simulink model "ControlSystem"  (R2026a)
settings: Solver=FixedStepDiscrete  FixedStep=1/200
undefined symbols (not defined in the file or in its folder): control, position, reversible_flags, timestamp, timestamp_sample, velocity
libraries: px4_lib x31
settings Model: Creator=jack  LastModifiedBy=jack
settings OptimizationCC: DefaultUnderspecifiedDataType=single
settings DebuggingCC: ParameterPrecisionLossMsg=none  UnnecessaryDatatypeConvMsg=warning
settings HardwareCC: ProdBitPerLong=64.0  ProdHWDeviceType=Intel->x86-64 (Linux 64)
settings SFSimCC: SimCustomHeaderCode="#include \"px4_simulink_api.h\""  SimUserSources=px4_simulink_api.cpp  SimTargetLang=C++
settings RTWCC: SystemTargetFile=ert.tlc  GenCodeOnly=on  PostCodeGenCommand=px4io.px4API.runPostCodeGen(buildInfo)  CustomHeaderCode="#include \"px4_simulink_api.h\""  DataTypeReplacement=CDataTypesFixedWidth  TargetLang=C++  Description=Embedded Coder
settings ERTTargetCC: ExtModeTransport=2.0  RootIOFormat=Structure reference  MaxIdInt64=INT64_MAX  MinIdInt64=INT64_MIN  MaxIdUint64=UINT64_MAX  MaxIdInt32=INT32_MAX  MinIdInt32=INT32_MIN  MaxIdUint32=UINT32_MAX  MaxIdInt16=INT16_MAX  MinIdInt16=INT16_MIN  MaxIdUint16=UINT16_MAX  MaxIdInt8=INT8_MAX  MinIdInt8=INT8_MIN  MaxIdUint8=UINT8_MAX  TargetLangStandard=C++14 (ISO)  CodeInterfacePackaging=C++ class  SubcomponentCodeInterfacePackaging=C++ class  ParenthesesLevel=Standards  CastingMode=Standards

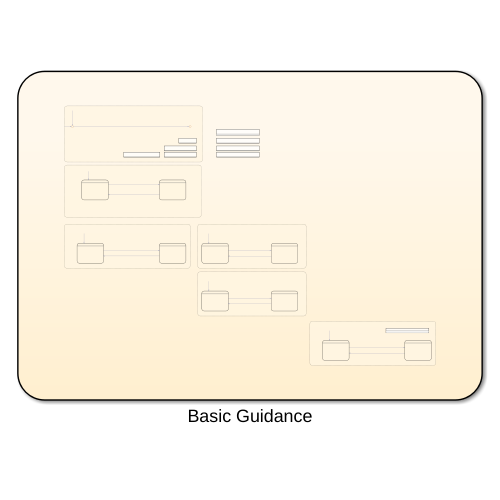
[thumbnail: Simulink's stored preview of the top-level diagram]
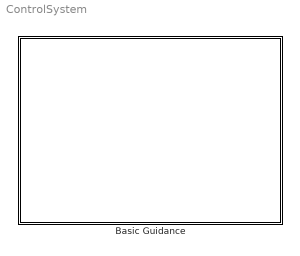
== system ControlSystem ==
  Basic Guidance : Stateflow chart  TreatAsAtomicUnit=on

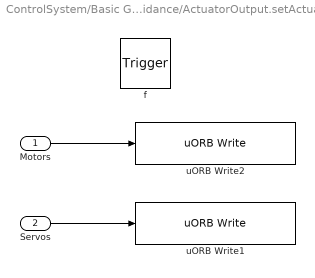
== system ControlSystem/Basic Guidance/ActuatorOutput.setActuators ==
  Motors : Inport  OutDataTypeStr=Bus: actuator_motors_s  PortDimensions=1
  Servos : Inport  Port=2  OutDataTypeStr=Bus: actuator_servos_s  PortDimensions=1
  f : TriggerPort  TriggerType=function-call  VariantControl=(inherit)
      settings: CopyFcn=Stateflow.SLINSF.SimulinkMan.removeBlockPreDeleteFcn  PreDeleteFcn=Stateflow.SLINSF.SimulinkMan.unsafePredeleteFcn
  uORB Write1 : px4_lib/uORB Write  uorb_topic=actuator_servos  uorb_variant=actuator_servos  sample_time=-1
  uORB Write2 : px4_lib/uORB Write  uorb_topic=actuator_motors  uorb_variant=actuator_motors  sample_time=-1
  wires:
  Motors/1 -> uORB Write2/1
  Servos/1 -> uORB Write1/1

== system ControlSystem/Basic Guidance/GuidanceRequestUpdate.Update.setGuidanceRequest ==
  GuidanceRequest : Inport  OutDataTypeStr=Bus: sim_guidance_request_s  PortDimensions=1
  f : TriggerPort  TriggerType=function-call  VariantControl=(inherit)
      settings: CopyFcn=Stateflow.SLINSF.SimulinkMan.removeBlockPreDeleteFcn  PreDeleteFcn=Stateflow.SLINSF.SimulinkMan.unsafePredeleteFcn
  uORB Write : px4_lib/uORB Write  uorb_topic=sim_guidance_request  uorb_variant=sim_guidance_request  sample_time=-1
  wires:
  GuidanceRequest/1 -> uORB Write/1

== system ControlSystem/Basic Guidance/InputProcessing.getGuidanceStatus ==
  f : TriggerPort  TriggerType=function-call  VariantControl=(inherit)
      settings: CopyFcn=Stateflow.SLINSF.SimulinkMan.removeBlockPreDeleteFcn  PreDeleteFcn=Stateflow.SLINSF.SimulinkMan.unsafePredeleteFcn
  uORB Read2 : px4_lib/uORB Read  uorb_topic=sim_guidance_status  uorb_variant=sim_guidance_status  sample_time=-1
  GuidanceStatus : Outport
  wires:
  uORB Read2/1 -> GuidanceStatus/1

== system ControlSystem/Basic Guidance/InputProcessing.getVehicleLandDetected ==
  f : TriggerPort  TriggerType=function-call  VariantControl=(inherit)
      settings: CopyFcn=Stateflow.SLINSF.SimulinkMan.removeBlockPreDeleteFcn  PreDeleteFcn=Stateflow.SLINSF.SimulinkMan.unsafePredeleteFcn
  uORB Read2 : px4_lib/uORB Read  uorb_topic=vehicle_land_detected  uorb_variant=vehicle_land_detected  sample_time=-1
  VehicleStatus : Outport
  wires:
  uORB Read2/1 -> VehicleStatus/1

== system ControlSystem/Basic Guidance/InputProcessing.getVehicleStatus ==
  f : TriggerPort  TriggerType=function-call  VariantControl=(inherit)
      settings: CopyFcn=Stateflow.SLINSF.SimulinkMan.removeBlockPreDeleteFcn  PreDeleteFcn=Stateflow.SLINSF.SimulinkMan.unsafePredeleteFcn
  uORB Read2 : px4_lib/uORB Read  uorb_topic=vehicle_status  uorb_variant=vehicle_status  sample_time=-1
  VehicleStatus : Outport
  wires:
  uORB Read2/1 -> VehicleStatus/1

== system ControlSystem/Basic Guidance/InputProcessing.isArmed ==
  f : TriggerPort  TriggerType=function-call  VariantControl=(inherit)
      settings: CopyFcn=Stateflow.SLINSF.SimulinkMan.removeBlockPreDeleteFcn  PreDeleteFcn=Stateflow.SLINSF.SimulinkMan.unsafePredeleteFcn
  Subsystem : Subsystem
  uORB Read3 : px4_lib/uORB Read  uorb_topic=actuator_armed  uorb_variant=actuator_armed  sample_time=-1
  Armed : Outport
  wires:
  uORB Read3/1 -> Subsystem/1(Actuator Armed)
  Subsystem/1(Armed) -> Armed/1

== system ControlSystem/Basic Guidance/OffboardControlModeUpdate.Update.setOffboardControlMode ==
  OffboardControlMode : Inport  OutDataTypeStr=Bus: offboard_control_mode_s  PortDimensions=1
  f : TriggerPort  TriggerType=function-call  VariantControl=(inherit)
      settings: CopyFcn=Stateflow.SLINSF.SimulinkMan.removeBlockPreDeleteFcn  PreDeleteFcn=Stateflow.SLINSF.SimulinkMan.unsafePredeleteFcn
  uORB Write2 : px4_lib/uORB Write  uorb_topic=offboard_control_mode  uorb_variant=offboard_control_mode  sample_time=-1
  wires:
  OffboardControlMode/1 -> uORB Write2/1

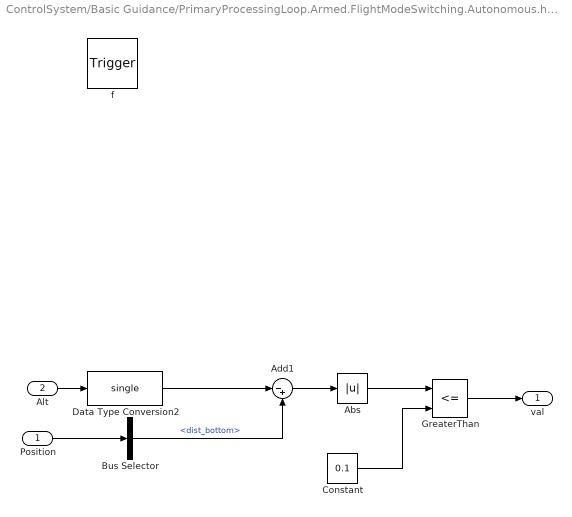
== system ControlSystem/Basic Guidance/PrimaryProcessingLoop.Armed.FlightModeSwitching.Autonomous.hasTakenOff ==
  Position : Inport  OutDataTypeStr=Bus: vehicle_local_position_s  PortDimensions=1
  Alt : Inport  Port=2  OutDataTypeStr=double  PortDimensions=1
  f : TriggerPort  TriggerType=function-call  VariantControl=(inherit)
      settings: CopyFcn=Stateflow.SLINSF.SimulinkMan.removeBlockPreDeleteFcn  PreDeleteFcn=Stateflow.SLINSF.SimulinkMan.unsafePredeleteFcn
  Abs : Abs  SaturateOnIntegerOverflow=off
  Add1 : Sum  Inputs=|-+
  Bus Selector : BusSelector  OutputSignals=dist_bottom
  Constant : Constant  Value=0.1
  Data Type Conversion2 : DataTypeConversion  OutDataTypeStr=single  SaturateOnIntegerOverflow=off  RndMeth=Floor
  GreaterThan : RelationalOperator  Operator=<=  OutDataTypeStr=boolean  RndMeth=Simplest  InputSameDT=off
  val : Outport  PortDimensions=1
  wires:
  Bus Selector/1 -> Add1/2  "<dist_bottom>"
  GreaterThan/1 -> val/1
  Position/1 -> Bus Selector/1
  Alt/1 -> Data Type Conversion2/1
  Data Type Conversion2/1 -> Add1/1
  Add1/1 -> Abs/1
  Constant/1 -> GreaterThan/2
  Abs/1 -> GreaterThan/1

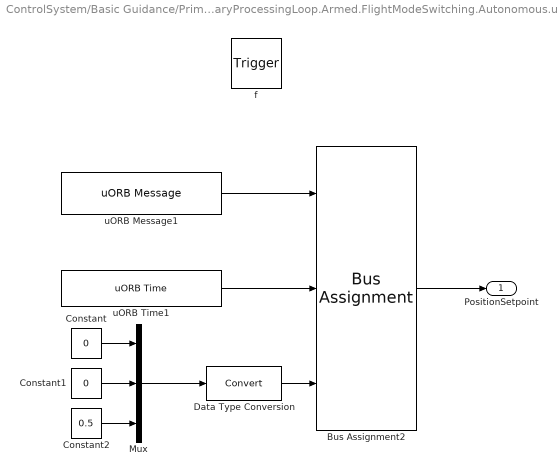
== system ControlSystem/Basic Guidance/PrimaryProcessingLoop.Armed.FlightModeSwitching.Autonomous.updateLand ==
  f : TriggerPort  TriggerType=function-call  VariantControl=(inherit)
      settings: CopyFcn=Stateflow.SLINSF.SimulinkMan.removeBlockPreDeleteFcn  PreDeleteFcn=Stateflow.SLINSF.SimulinkMan.unsafePredeleteFcn
  Bus Assignment2 : BusAssignment  AssignedSignals=timestamp,velocity
  Constant : Constant  Value=0
  Constant1 : Constant  Value=0
  Constant2 : Constant  Value=0.5
  Data Type Conversion : DataTypeConversion  SaturateOnIntegerOverflow=off  RndMeth=Floor
  Mux : Mux  Inputs=3
  uORB Message1 : px4_lib/uORB Message  uorb_topic=trajectory_setpoint  uorb_variant=trajectory_setpoint  init_value=NaN  sample_time=-1
  uORB Time1 : px4_lib/uORB Time  sample_time=-1
  PositionSetpoint : Outport  OutDataTypeStr=Bus: trajectory_setpoint_s  PortDimensions=1
  wires:
  uORB Message1/1 -> Bus Assignment2/1
  uORB Time1/1 -> Bus Assignment2/2
  Bus Assignment2/1 -> PositionSetpoint/1
  Mux/1 -> Data Type Conversion/1
  Constant2/1 -> Mux/3
  Constant1/1 -> Mux/2
  Constant/1 -> Mux/1
  Data Type Conversion/1 -> Bus Assignment2/3

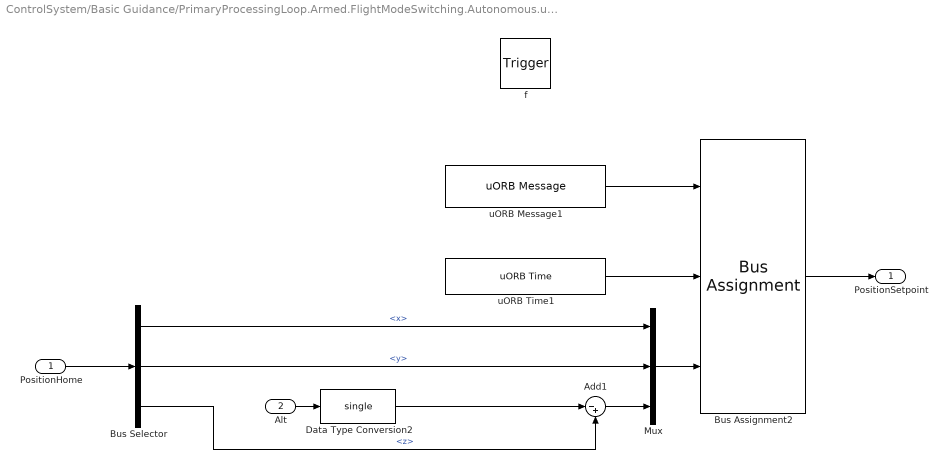
== system ControlSystem/Basic Guidance/PrimaryProcessingLoop.Armed.FlightModeSwitching.Autonomous.updateTakeoff ==
  PositionHome : Inport  OutDataTypeStr=Bus: vehicle_local_position_s  PortDimensions=1
  Alt : Inport  Port=2  OutDataTypeStr=double  PortDimensions=1
  f : TriggerPort  TriggerType=function-call  VariantControl=(inherit)
      settings: CopyFcn=Stateflow.SLINSF.SimulinkMan.removeBlockPreDeleteFcn  PreDeleteFcn=Stateflow.SLINSF.SimulinkMan.unsafePredeleteFcn
  Add1 : Sum  Inputs=|-+
  Bus Assignment2 : BusAssignment  AssignedSignals=timestamp,position
  Bus Selector : BusSelector  OutputSignals=x,y,z
  Data Type Conversion2 : DataTypeConversion  OutDataTypeStr=single  SaturateOnIntegerOverflow=off  RndMeth=Floor
  Mux : Mux  Inputs=3
  uORB Message1 : px4_lib/uORB Message  uorb_topic=trajectory_setpoint  uorb_variant=trajectory_setpoint  init_value=NaN  sample_time=-1
  uORB Time1 : px4_lib/uORB Time  sample_time=-1
  PositionSetpoint : Outport  OutDataTypeStr=Bus: trajectory_setpoint_s  PortDimensions=1
  wires:
  uORB Message1/1 -> Bus Assignment2/1
  uORB Time1/1 -> Bus Assignment2/2
  Bus Selector/3 -> Add1/2  "<z>"
  Bus Assignment2/1 -> PositionSetpoint/1
  PositionHome/1 -> Bus Selector/1
  Alt/1 -> Data Type Conversion2/1
  Data Type Conversion2/1 -> Add1/1
  Add1/1 -> Mux/3
  Bus Selector/2 -> Mux/2  "<y>"
  Bus Selector/1 -> Mux/1  "<x>"
  Mux/1 -> Bus Assignment2/3

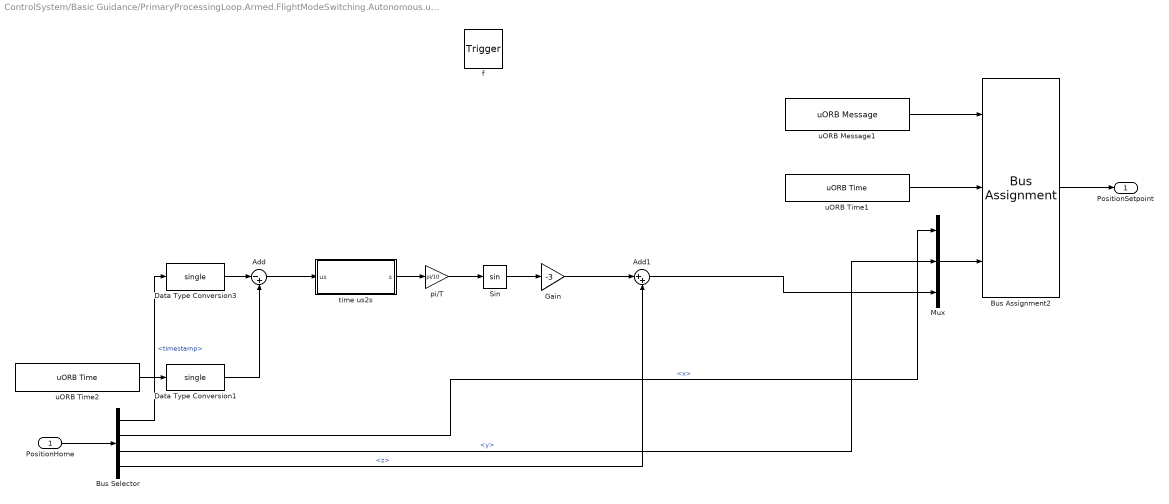
== system ControlSystem/Basic Guidance/PrimaryProcessingLoop.Armed.FlightModeSwitching.Autonomous.updateTrajectory ==
  PositionHome : Inport  OutDataTypeStr=Bus: vehicle_local_position_s  PortDimensions=1
  f : TriggerPort  TriggerType=function-call  VariantControl=(inherit)
      settings: CopyFcn=Stateflow.SLINSF.SimulinkMan.removeBlockPreDeleteFcn  PreDeleteFcn=Stateflow.SLINSF.SimulinkMan.unsafePredeleteFcn
  Add : Sum  Inputs=|-+
  Add1 : Sum  Inputs=|++
  Bus Assignment2 : BusAssignment  AssignedSignals=timestamp,position
  Bus Selector : BusSelector  OutputSignals=timestamp,x,y,z
  Data Type Conversion1 : DataTypeConversion  OutDataTypeStr=single  SaturateOnIntegerOverflow=off  RndMeth=Floor
  Data Type Conversion3 : DataTypeConversion  OutDataTypeStr=single  SaturateOnIntegerOverflow=off  RndMeth=Floor
  Gain : Gain  Gain=-3  ParamDataTypeStr=single
  Mux : Mux  Inputs=3
  Sin : Trigonometry  OutputSignalType=real
  pi/T : Gain  Gain=pi/10  ParamDataTypeStr=single
  time us2s : Subsystem
  uORB Message1 : px4_lib/uORB Message  uorb_topic=trajectory_setpoint  uorb_variant=trajectory_setpoint  init_value=NaN  sample_time=-1
  uORB Time1 : px4_lib/uORB Time  sample_time=-1
  uORB Time2 : px4_lib/uORB Time  sample_time=-1
  PositionSetpoint : Outport  OutDataTypeStr=Bus: trajectory_setpoint_s  PortDimensions=1
  wires:
  uORB Time2/1 -> Data Type Conversion1/1
  uORB Message1/1 -> Bus Assignment2/1
  Bus Selector/1 -> Data Type Conversion3/1  "<timestamp>"
  pi/T/1 -> Sin/1
  uORB Time1/1 -> Bus Assignment2/2
  Add/1 -> time us2s/1(us)
  time us2s/1(s) -> pi/T/1
  Sin/1 -> Gain/1
  Bus Selector/4 -> Add1/2  "<z>"
  Bus Assignment2/1 -> PositionSetpoint/1
  PositionHome/1 -> Bus Selector/1
  Data Type Conversion1/1 -> Add/2
  Data Type Conversion3/1 -> Add/1
  Gain/1 -> Add1/1
  Bus Selector/2 -> Mux/1  "<x>"
  Bus Selector/3 -> Mux/2  "<y>"
  Add1/1 -> Mux/3
  Mux/1 -> Bus Assignment2/3

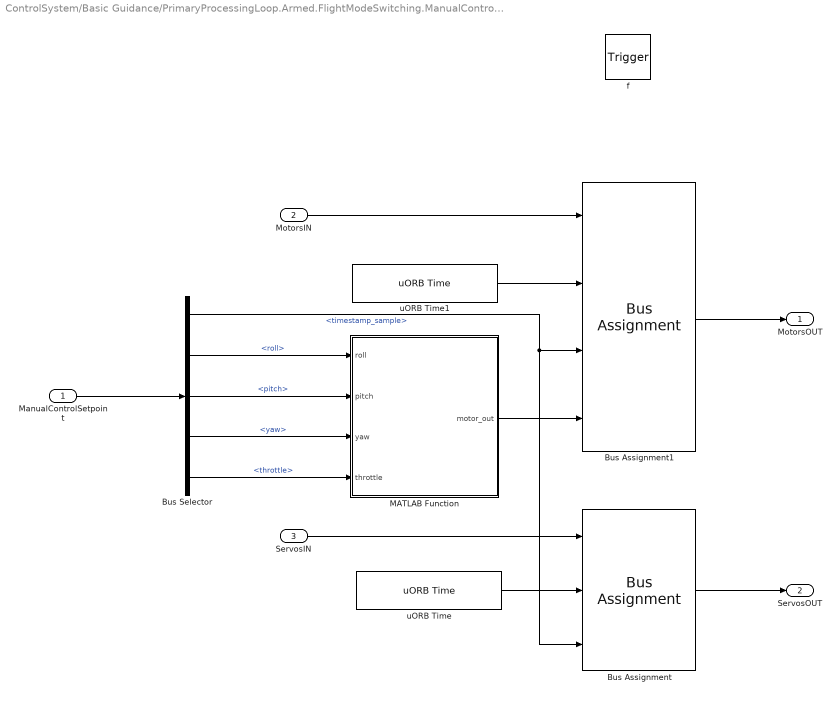
== system ControlSystem/Basic Guidance/PrimaryProcessingLoop.Armed.FlightModeSwitching.ManualControl.updateManualControl ==
  ManualControlSetpoint : Inport  OutDataTypeStr=Bus: manual_control_setpoint_s  PortDimensions=1
  MotorsIN : Inport  Port=2  OutDataTypeStr=Bus: actuator_motors_s  PortDimensions=1
  ServosIN : Inport  Port=3  OutDataTypeStr=Bus: actuator_servos_s  PortDimensions=1
  f : TriggerPort  TriggerType=function-call  VariantControl=(inherit)
      settings: CopyFcn=Stateflow.SLINSF.SimulinkMan.removeBlockPreDeleteFcn  PreDeleteFcn=Stateflow.SLINSF.SimulinkMan.unsafePredeleteFcn
  Bus Assignment : BusAssignment  AssignedSignals=timestamp,timestamp_sample
  Bus Assignment1 : BusAssignment  AssignedSignals=timestamp,timestamp_sample,control
  Bus Selector : BusSelector  OutputSignals=timestamp_sample,roll,pitch,yaw,throttle
  MATLAB Function : MATLAB Function  TreatAsAtomicUnit=on
  uORB Time : px4_lib/uORB Time  sample_time=-1
  uORB Time1 : px4_lib/uORB Time  sample_time=-1
  MotorsOUT : Outport  OutDataTypeStr=Bus: actuator_motors_s  PortDimensions=1
  ServosOUT : Outport  Port=2  OutDataTypeStr=Bus: actuator_servos_s  PortDimensions=1
  wires:
  ServosIN/1 -> Bus Assignment/1
  Bus Assignment/1 -> ServosOUT/1
  uORB Time/1 -> Bus Assignment/2
  MotorsIN/1 -> Bus Assignment1/1
  Bus Assignment1/1 -> MotorsOUT/1
  MATLAB Function/1(motor_out) -> Bus Assignment1/4
  ManualControlSetpoint/1 -> Bus Selector/1
  Bus Selector/5 -> MATLAB Function/4(throttle)  "<throttle>"
  Bus Selector/4 -> MATLAB Function/3(yaw)  "<yaw>"
  Bus Selector/3 -> MATLAB Function/2(pitch)  "<pitch>"
  Bus Selector/2 -> MATLAB Function/1(roll)  "<roll>"
  uORB Time1/1 -> Bus Assignment1/2
  Bus Selector/1 -> Bus Assignment1/3, Bus Assignment/3  "<timestamp_sample>"

== system ControlSystem/Basic Guidance/PrimaryProcessingLoop.Armed.FlightModeSwitching.getPosition ==
  f : TriggerPort  TriggerType=function-call  VariantControl=(inherit)
      settings: CopyFcn=Stateflow.SLINSF.SimulinkMan.removeBlockPreDeleteFcn  PreDeleteFcn=Stateflow.SLINSF.SimulinkMan.unsafePredeleteFcn
  uORB Read2 : px4_lib/uORB Read  uorb_topic=vehicle_local_position  uorb_variant=vehicle_local_position  sample_time=-1
  Position : Outport
  wires:
  uORB Read2/1 -> Position/1

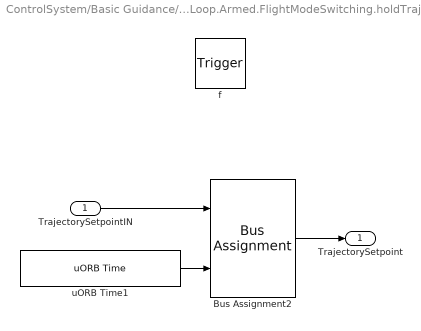
== system ControlSystem/Basic Guidance/PrimaryProcessingLoop.Armed.FlightModeSwitching.holdTrajectorySetpoint ==
  TrajectorySetpointIN : Inport  OutDataTypeStr=Bus: trajectory_setpoint_s  PortDimensions=1
  f : TriggerPort  TriggerType=function-call  VariantControl=(inherit)
      settings: CopyFcn=Stateflow.SLINSF.SimulinkMan.removeBlockPreDeleteFcn  PreDeleteFcn=Stateflow.SLINSF.SimulinkMan.unsafePredeleteFcn
  Bus Assignment2 : BusAssignment  AssignedSignals=timestamp
  uORB Time1 : px4_lib/uORB Time  sample_time=-1
  TrajectorySetpoint : Outport  OutDataTypeStr=Bus: trajectory_setpoint_s  PortDimensions=1
  wires:
  Bus Assignment2/1 -> TrajectorySetpoint/1
  uORB Time1/1 -> Bus Assignment2/2
  TrajectorySetpointIN/1 -> Bus Assignment2/1

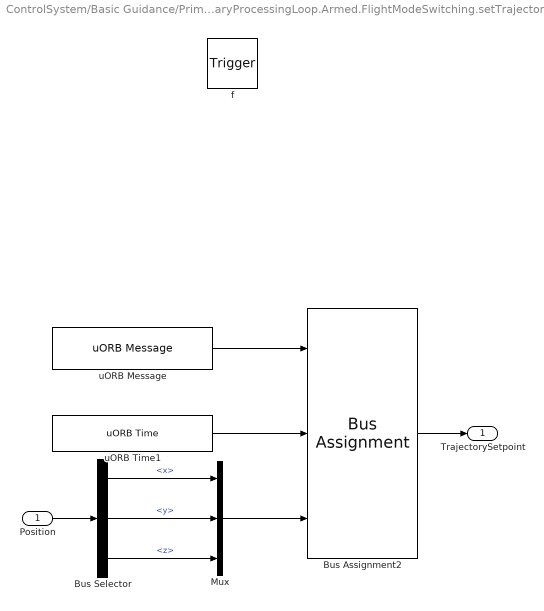
== system ControlSystem/Basic Guidance/PrimaryProcessingLoop.Armed.FlightModeSwitching.setTrajectorySetpoint ==
  Position : Inport  OutDataTypeStr=Bus: vehicle_local_position_s  PortDimensions=1
  f : TriggerPort  TriggerType=function-call  VariantControl=(inherit)
      settings: CopyFcn=Stateflow.SLINSF.SimulinkMan.removeBlockPreDeleteFcn  PreDeleteFcn=Stateflow.SLINSF.SimulinkMan.unsafePredeleteFcn
  Bus Assignment2 : BusAssignment  AssignedSignals=timestamp,position
  Bus Selector : BusSelector  OutputSignals=x,y,z
  Mux : Mux  Inputs=3
  uORB Message : px4_lib/uORB Message  uorb_topic=trajectory_setpoint  uorb_variant=trajectory_setpoint  init_value=NaN  sample_time=-1
  uORB Time1 : px4_lib/uORB Time  sample_time=-1
  TrajectorySetpoint : Outport  OutDataTypeStr=Bus: trajectory_setpoint_s  PortDimensions=1
  wires:
  uORB Message/1 -> Bus Assignment2/1
  Bus Assignment2/1 -> TrajectorySetpoint/1
  uORB Time1/1 -> Bus Assignment2/2
  Position/1 -> Bus Selector/1
  Bus Selector/3 -> Mux/3  "<z>"
  Bus Selector/2 -> Mux/2  "<y>"
  Bus Selector/1 -> Mux/1  "<x>"
  Mux/1 -> Bus Assignment2/3

== system ControlSystem/Basic Guidance/SetpointTrajectoryUpdate.Update.setTrajectorySetpoint ==
  TrajectorySetpoint : Inport  OutDataTypeStr=Bus: trajectory_setpoint_s  PortDimensions=1
  f : TriggerPort  TriggerType=function-call  VariantControl=(inherit)
      settings: CopyFcn=Stateflow.SLINSF.SimulinkMan.removeBlockPreDeleteFcn  PreDeleteFcn=Stateflow.SLINSF.SimulinkMan.unsafePredeleteFcn
  uORB Write1 : px4_lib/uORB Write  uorb_topic=trajectory_setpoint  uorb_variant=trajectory_setpoint  sample_time=-1
  wires:
  TrajectorySetpoint/1 -> uORB Write1/1

== system ControlSystem/Basic Guidance/getManualControl ==
  f : TriggerPort  TriggerType=function-call  VariantControl=(inherit)
      settings: CopyFcn=Stateflow.SLINSF.SimulinkMan.removeBlockPreDeleteFcn  PreDeleteFcn=Stateflow.SLINSF.SimulinkMan.unsafePredeleteFcn
  uORB Read2 : px4_lib/uORB Read  uorb_topic=manual_control_setpoint  uorb_variant=manual_control_setpoint  sample_time=-1
  ManualControlSetpoint : Outport
  wires:
  uORB Read2/1 -> ManualControlSetpoint/1

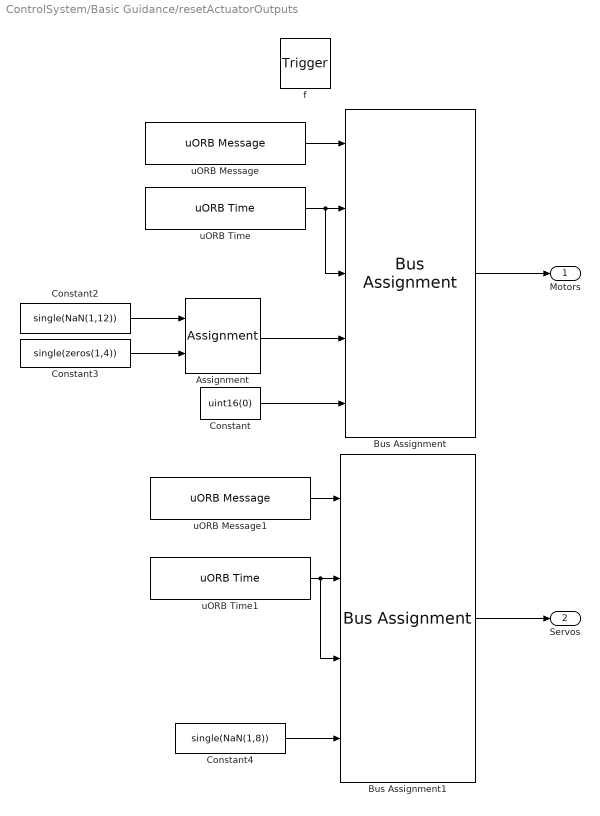
== system ControlSystem/Basic Guidance/resetActuatorOutputs ==
  f : TriggerPort  TriggerType=function-call  VariantControl=(inherit)
      settings: CopyFcn=Stateflow.SLINSF.SimulinkMan.removeBlockPreDeleteFcn  PreDeleteFcn=Stateflow.SLINSF.SimulinkMan.unsafePredeleteFcn
  Assignment : Assignment  DiagnosticForDimensions=Warning  IndexOptions=Index vector (dialog)  Indices=1:4  OutputSizes=1
  Bus Assignment : BusAssignment  AssignedSignals=timestamp,timestamp_sample,control,reversible_flags
  Bus Assignment1 : BusAssignment  AssignedSignals=timestamp,timestamp_sample,control
  Constant : Constant  Value=uint16(0)
  Constant2 : Constant  Value=single(NaN(1,12))
  Constant3 : Constant  Value=single(zeros(1,4))
  Constant4 : Constant  Value=single(NaN(1,8))
  uORB Message : px4_lib/uORB Message  uorb_topic=actuator_motors  uorb_variant=actuator_motors  init_value=NaN  sample_time=-1
  uORB Message1 : px4_lib/uORB Message  uorb_topic=actuator_servos  uorb_variant=actuator_servos  init_value=NaN  sample_time=-1
  uORB Time : px4_lib/uORB Time  sample_time=-1
  uORB Time1 : px4_lib/uORB Time  sample_time=-1
  Motors : Outport
  Servos : Outport  Port=2
  wires:
  Bus Assignment/1 -> Motors/1
  uORB Message/1 -> Bus Assignment/1
  uORB Time/1 -> Bus Assignment/3, Bus Assignment/2
  uORB Time1/1 -> Bus Assignment1/3, Bus Assignment1/2
  uORB Message1/1 -> Bus Assignment1/1
  Bus Assignment1/1 -> Servos/1
  Constant/1 -> Bus Assignment/5
  Assignment/1 -> Bus Assignment/4
  Constant3/1 -> Assignment/2
  Constant2/1 -> Assignment/1
  Constant4/1 -> Bus Assignment1/4

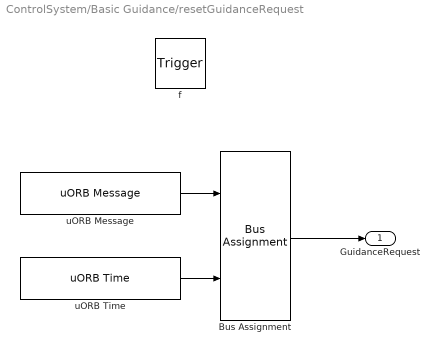
== system ControlSystem/Basic Guidance/resetGuidanceRequest ==
  f : TriggerPort  TriggerType=function-call  VariantControl=(inherit)
      settings: CopyFcn=Stateflow.SLINSF.SimulinkMan.removeBlockPreDeleteFcn  PreDeleteFcn=Stateflow.SLINSF.SimulinkMan.unsafePredeleteFcn
  Bus Assignment : BusAssignment  AssignedSignals=timestamp
  uORB Message : px4_lib/uORB Message  uorb_topic=sim_guidance_request  uorb_variant=sim_guidance_request  init_value=0  sample_time=-1
  uORB Time : px4_lib/uORB Time  sample_time=-1
  GuidanceRequest : Outport
  wires:
  Bus Assignment/1 -> GuidanceRequest/1
  uORB Message/1 -> Bus Assignment/1
  uORB Time/1 -> Bus Assignment/2

== system ControlSystem/Basic Guidance/resetOffboardControlMode ==
  f : TriggerPort  TriggerType=function-call  VariantControl=(inherit)
      settings: CopyFcn=Stateflow.SLINSF.SimulinkMan.removeBlockPreDeleteFcn  PreDeleteFcn=Stateflow.SLINSF.SimulinkMan.unsafePredeleteFcn
  Bus Assignment : BusAssignment  AssignedSignals=timestamp
  uORB Message : px4_lib/uORB Message  uorb_topic=offboard_control_mode  uorb_variant=offboard_control_mode  init_value=0  sample_time=-1
  uORB Time : px4_lib/uORB Time  sample_time=-1
  OffboardControlMode : Outport
  wires:
  uORB Message/1 -> Bus Assignment/1
  Bus Assignment/1 -> OffboardControlMode/1
  uORB Time/1 -> Bus Assignment/2

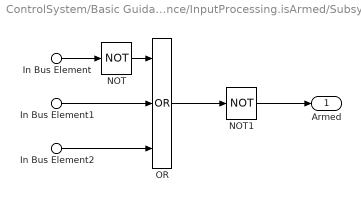
== system ControlSystem/Basic Guidance/InputProcessing.isArmed/Subsystem ==
  In Bus Element : Inport  PortName=Actuator Armed  Element=armed
  In Bus Element1 : Inport  PortName=Actuator Armed  Element=lockdown
  In Bus Element2 : Inport  PortName=Actuator Armed  Element=in_esc_calibration_mode
  NOT : Logic  Operator=NOT  IconShape=distinctive  AllPortsSameDT=off  OutDataTypeStr=boolean
  NOT1 : Logic  Operator=NOT  IconShape=distinctive  AllPortsSameDT=off  OutDataTypeStr=boolean
  OR : Logic  Operator=OR  Inputs=3  IconShape=distinctive  AllPortsSameDT=off  OutDataTypeStr=boolean
  Armed : Outport
  wires:
  NOT1/1 -> Armed/1
  In Bus Element/1 -> NOT/1
  In Bus Element1/1 -> OR/2
  In Bus Element2/1 -> OR/3
  NOT/1 -> OR/1
  OR/1 -> NOT1/1

== system ControlSystem/Basic Guidance/PrimaryProcessingLoop.Armed.FlightModeSwitching.Autonomous.updateTrajectory/time us2s ==
  us : Inport
  us to s : Gain  Gain=single(1E-6)  ParamDataTypeStr=single
  s : Outport
  wires:
  us/1 -> us to s/1
  us to s/1 -> s/1

== matlab function ControlSystem/Basic Guidance/PrimaryProcessingLoop.Armed.FlightModeSwitching.ManualControl.updateManualControl/MATLAB Function ==
  data: motor_out output; roll input; pitch input; yaw input; throttle input
function motor_out = fcn(roll, pitch, yaw, throttle)
motor_out = repmat(single(NaN), [1,12]);
Thrust_Base = (throttle + 1.0) / 2.0;

% Scale down attitude sticks for safe bench/simulation testing
R = roll  * 0.01;
P = pitch * 0.01;
Y = yaw   * 0.01;
T = Thrust_Base;

% Quad-X Direct Motor Mapping (Normalized 0.0 to 1.0)
motor_out(1) = T - R - P + Y;  % Front Right (CCW)
motor_out(2) = T + R + P + Y;  % Back Left (CCW)
motor_out(3) = T + R - P - Y;  % Front Left (CW)
motor_out(4) = T - R + P - Y;  % Back Right (CW)

for i = 1:4
    motor_out(i) = saturate(motor_out(i), 0, 1);
end
end


function out = saturate(in, min_val, max_val)
out = max(min(in, max_val), min_val);
end

== stateflow chart ControlSystem/Basic Guidance ==
  settings: updateMethod=DISCRETE  sampleTime=1/200
  state InputProcessing [parallel]
    settings: executionOrder=1
    state Armed = isArmed [function]
    state GuidanceStatus = getGuidanceStatus [function]
    state VehicleStatus = getVehicleLandDetected [function]
    state VehicleStatus = getVehicleStatus [function]
    (default) -> (junction 352) : {
        | GuidanceRequest = resetGuidanceRequest();
        | OffboardControlMode = resetOffboardControlMode();
        | [MotorOutputs, ServoOutputs] = resetActuatorOutputs();
        | }
    InputProcessing -> (junction 352)
    (junction 352) -> (junction 353) : {
        | ArmedRequest = isArmed();
        | GuidanceStatus = getGuidanceStatus();
        | VehicleStatus = getVehicleStatus();
        | VehicleLandDetected = getVehicleLandDetected();
        | ManualControlSetpoint = getManualControl();
        | }
  state ManualControlSetpoint = getManualControl [function]
  state [Motors,Servos] = resetActuatorOutputs [function]
  state GuidanceRequest = resetGuidanceRequest [function]
  state OffboardControlMode = resetOffboardControlMode [function]
  state PrimaryProcessingLoop [parallel]
    settings: executionOrder=2
    state Disarmed
      state Idle
      (default) -> PrimaryProcessingLoop.Disarmed.Idle : {
          | pauseSetpointTrajectoryUpdate = true;
          | }
      PrimaryProcessingLoop.Disarmed.Idle -> (junction 133) : [GuidanceStatus.started && ~GuidanceStatus.finished]
          | {GuidanceRequest.stop = true;}
      (junction 133) -> PrimaryProcessingLoop.Disarmed.Idle
    state Armed
      state FlightModeSwitching [parallel]
        settings: executionOrder=1
        state PositionHold
          state UpdateCurrentState
            entry, during:
            OffboardControlMode.position = true;
            TrajectorySetpoint = holdTrajectorySetpoint(TrajectorySetpoint);
          (default) -> UpdateCurrentState : {
              | pauseSetpointTrajectoryUpdate = false;
              | GuidanceRequest.stop = true;
              | }
        state PositionControl
          (default) -> (junction 501) : {
              | pauseSetpointTrajectoryUpdate = true;
              | GuidanceRequest.stop = true;
              | }
        state ManualControl
          state [MotorsOUT, ServosOUT] = updateManualControl(ManualControlSetpoint, MotorsIN, ServosIN) [function]
          (default) -> (junction 502) : {
              | pauseSetpointTrajectoryUpdate = true;
              | GuidanceRequest.stop = true;
              | }
          ManualControl -> (junction 502) [order 1]
          (junction 502) -> (junction 504) : {[MotorOutputs, ServoOutputs] = updateManualControl(ManualControlSetpoint, MotorOutputs, ServoOutputs)}
        state Autonomous
          state Landed
            entry:
            takeoff_altitude = 10;
            PositionHome = getPosition();
            GuidanceRequest.reset = true;
            GuidanceRequest.start = true;
            entry, during:
            OffboardControlMode.position = true;
            TrajectorySetpoint = setTrajectorySetpoint(PositionHome);
          state Takeoff
            entry:
            entry, during:
            OffboardControlMode.position = true;
            TrajectorySetpoint = updateTakeoff(PositionHome, takeoff_altitude);
          state Flying
            entry:
            GuidanceRequest.start_execution = true;
            pauseSetpointTrajectoryUpdate = true;
            entry, during:
            OffboardControlMode.position = true;
            OffboardControlMode.velocity = true;
            OffboardControlMode.acceleration = true;
          state Land
            entry:
            pauseSetpointTrajectoryUpdate = false;
            entry, during:
            OffboardControlMode.velocity = true;
            TrajectorySetpoint = updateLand();
          state PositionSetpoint = updateTrajectory(PositionHome) [function] [commented out]
          state val = hasTakenOff(Position,Alt) [function]
          state PositionSetpoint = updateTakeoff(PositionHome, Alt) [function]
          state PositionSetpoint = updateLand [function]
          (default) -> Landed : {pauseSetpointTrajectoryUpdate = false;}
          Takeoff -> Flying [order 1] : [hasTakenOff(getPosition(), takeoff_altitude) && ~VehicleLandDetected.landed]
              | {GuidanceRequest.set_home = true;}
          Landed -> Takeoff : [GuidanceStatus.loaded && GuidanceStatus.started]
          Flying -> Land [order 1] : [GuidanceStatus.finished]
          (junction 258) -> Landed : [after(2,sec)]{pauseSetpointTrajectoryUpdate = false;}
          Takeoff -> (junction 259) [order 2] : [VehicleLandDetected.landed]
          Flying -> (junction 260) [order 2] : [VehicleLandDetected.landed]
          Land -> (junction 450) : [VehicleLandDetected.landed]
          (junction 259) -> (junction 258)
          (junction 260) -> (junction 259)
          (junction 450) -> (junction 260)
        state TrajectorySetpoint = holdTrajectorySetpoint(TrajectorySetpointIN) [function]
        state Position = getPosition [function]
        state TrajectorySetpoint = setTrajectorySetpoint(Position) [function]
        (default) -> PositionHold : {
            | TrajectorySetpoint = setTrajectorySetpoint(getPosition());
            | pauseSetpointTrajectoryUpdate = true;
            | }
        (junction 381) -> (junction 377)
        (junction 377) -> (junction 148)
        (junction 379) -> (junction 381)
        (junction 148) -> (junction 374) [order 2]
        (junction 148) -> (junction 372) [order 3]
        (junction 148) -> ManualControl [order 4] : [VehicleStatus.nav_state == px4io.enums.vehicle_status.NAVIGATION_STATE_MANUAL]
        (junction 374) -> PositionHold : [VehicleStatus.nav_state == px4io.enums.vehicle_status.NAVIGATION_STATE_AUTO_LOITER]
        (junction 148) -> PositionControl [order 1] : [VehicleStatus.nav_state == px4io.enums.vehicle_status.NAVIGATION_STATE_POSCTL]
        (junction 372) -> Autonomous : [VehicleStatus.nav_state == px4io.enums.vehicle_status.NAVIGATION_STATE_OFFBOARD]
        ManualControl -> (junction 508) [order 1] : [VehicleStatus.nav_state ~= px4io.enums.vehicle_status.NAVIGATION_STATE_MANUAL]
        PositionHold -> (junction 370) : [VehicleStatus.nav_state ~= px4io.enums.vehicle_status.NAVIGATION_STATE_AUTO_LOITER]
        PositionControl -> (junction 367) : [VehicleStatus.nav_state ~= px4io.enums.vehicle_status.NAVIGATION_STATE_POSCTL]
        Autonomous -> (junction 368) : [VehicleStatus.nav_state ~= px4io.enums.vehicle_status.NAVIGATION_STATE_OFFBOARD]
        (junction 370) -> (junction 367)
        (junction 368) -> (junction 379)
        (junction 367) -> (junction 508)
        (junction 508) -> (junction 368)
    (default) -> PrimaryProcessingLoop.Disarmed
    PrimaryProcessingLoop.Disarmed -> Armed : [ArmedRequest]
    Armed -> PrimaryProcessingLoop.Disarmed : [~ArmedRequest]
  state GuidanceRequestUpdate [parallel]
    settings: executionOrder=3
    state Idle
      (default) -> (junction 228) : {GuidanceRequest = resetGuidanceRequest();}
    state Update
      state setGuidanceRequest(GuidanceRequest) [function]
      (default) -> (junction 231) : {setGuidanceRequest(GuidanceRequest);}
    (default) -> GuidanceRequestUpdate.Idle
    GuidanceRequestUpdate.Idle -> GuidanceRequestUpdate.Update : [
        | GuidanceRequest.start ...
        | || GuidanceRequest.stop ...
        | || GuidanceRequest.reset ...
        | || GuidanceRequest.set_home ...
        | || GuidanceRequest.start_execution
        | ]
    GuidanceRequestUpdate.Update -> GuidanceRequestUpdate.Idle
  state SetpointTrajectoryUpdate [parallel]
    settings: executionOrder=4
    state Idle
      (default) -> (junction 398)
    state Update
      state setTrajectorySetpoint(TrajectorySetpoint) [function]
      (default) -> (junction 402) : {
          | setTrajectorySetpoint(TrajectorySetpoint);
          | }
    (default) -> SetpointTrajectoryUpdate.Idle
    SetpointTrajectoryUpdate.Idle -> SetpointTrajectoryUpdate.Update : [~pauseSetpointTrajectoryUpdate]
    SetpointTrajectoryUpdate.Update -> SetpointTrajectoryUpdate.Idle
  state OffboardControlModeUpdate [parallel]
    settings: executionOrder=5
    state Idle
      (default) -> (junction 441) : {OffboardControlMode = resetOffboardControlMode();}
    state Update
      state setOffboardControlMode(OffboardControlMode) [function]
      (default) -> (junction 433) : {
          | setOffboardControlMode(OffboardControlMode);
          | }
    (default) -> OffboardControlModeUpdate.Idle
    OffboardControlModeUpdate.Idle -> OffboardControlModeUpdate.Update : [
        | OffboardControlMode.position || ...
        | OffboardControlMode.velocity || ...
        | OffboardControlMode.acceleration || ...
        | OffboardControlMode.attitude || ...
        | OffboardControlMode.body_rate || ...
        | OffboardControlMode.thrust_and_torque || ...
        | OffboardControlMode.direct_actuator
        | ]
    OffboardControlModeUpdate.Update -> OffboardControlModeUpdate.Idle
  state ActuatorOutput [parallel]
    settings: executionOrder=6
    state setActuators(Motors, Servos) [function]
    state Disarmed
      (default) -> (junction 462) : {[MotorOutputs, ServoOutputs] = resetActuatorOutputs();}
      ActuatorOutput.Disarmed -> (junction 462) [order 1]
      (junction 462) -> (junction 470) : {setActuators(MotorOutputs, ServoOutputs)}
    state Update
      (default) -> (junction 456)
      ActuatorOutput.Update -> (junction 456) [order 1]
      (junction 456) -> (junction 479) : {setActuators(MotorOutputs, ServoOutputs)}
    (default) -> ActuatorOutput.Disarmed
    ActuatorOutput.Disarmed -> ActuatorOutput.Update [order 1] : [in(PrimaryProcessingLoop.Armed)]
    ActuatorOutput.Update -> ActuatorOutput.Disarmed [order 1] : [in(PrimaryProcessingLoop.Disarmed)]
  data: Armed function_output; GuidanceStatus function_output; VehicleStatus function_output; VehicleStatus function_output; ManualControlSetpoint function_output; Motors function_output; Servos function_output; GuidanceRequest function_output; OffboardControlMode function_output; ManualControlSetpoint function_input Bus: manual_control_setpoint_s size=1; MotorsOUT function_output Bus: actuator_motors_s size=1; ServosOUT function_output Bus: actuator_servos_s size=1; MotorsIN function_input Bus: actuator_motors_s size=1; ServosIN function_input Bus: actuator_servos_s size=1; PositionHome function_input double size=1; PositionSetpoint function_output double size=1; Position function_input Bus: vehicle_local_position_s size=1; val function_output size=1; Alt function_input double size=1; PositionHome function_input Bus: vehicle_local_position_s size=1; PositionSetpoint function_output Bus: trajectory_setpoint_s size=1; Alt function_input double size=1; PositionSetpoint function_output Bus: trajectory_setpoint_s size=1; TrajectorySetpoint function_output Bus: trajectory_setpoint_s size=1; TrajectorySetpointIN function_input Bus: trajectory_setpoint_s size=1; Position function_output; TrajectorySetpoint function_output Bus: trajectory_setpoint_s size=1; Position function_input Bus: vehicle_local_position_s size=1; GuidanceRequest function_input Bus: sim_guidance_request_s size=1; TrajectorySetpoint function_input Bus: trajectory_setpoint_s size=1; OffboardControlMode function_input Bus: offboard_control_mode_s size=1; Motors function_input Bus: actuator_motors_s size=1; Servos function_input Bus: actuator_servos_s size=1; PositionHome local Bus: vehicle_local_position_s size=1; takeoff_altitude local; GuidanceStatus local Bus: sim_guidance_status_s size=1; GuidanceRequest local Bus: sim_guidance_request_s size=1; ArmedRequest local boolean size=1 =false; OffboardControlMode local Bus: offboard_control_mode_s size=1; VehicleStatus local Bus: vehicle_status_s size=1; TrajectorySetpoint local Bus: trajectory_setpoint_s size=1; pauseSetpointTrajectoryUpdate local boolean size=1 =true; VehicleLandDetected local Bus: vehicle_land_detected_s size=1; ServoOutputs local Bus: actuator_servos_s size=1; MotorOutputs local Bus: actuator_motors_s size=1; ManualControlSetpoint local Bus: manual_control_setpoint_s size=1
